simulink model "L4_sim1"  (R2024b)
settings: Solver=VariableStepAuto  StartTime=0.0  StopTime=100  RelTol=1e-3
values from neighbouring files (symbols this model uses):
  A_0 = eye(3)    [Task1.m]
  I = diag([Ix, Iy, Iz])    [Task1.m]    (also in Task3.m)
  orthonormalize = 0    [Task1.m]
  w_0 = [0.45, 0.52, 0.55]'    [Task1.m]    (also in Task3.m = [0.3, 0.15, 0.6]')
libraries: matrix_library x1
settings Model: Creator=alejandromunozvazquez  LastModifiedBy=alejandromunozvazquez

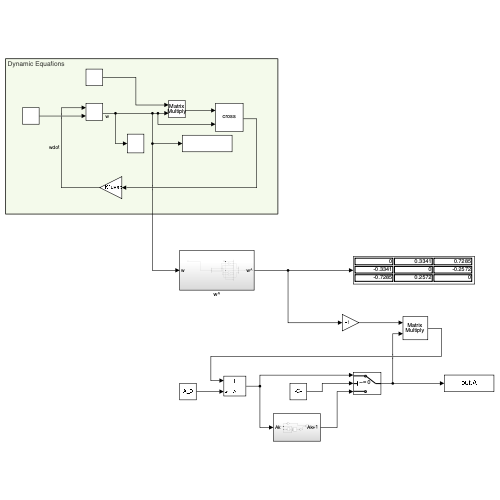
[thumbnail: Simulink's stored preview of the top-level diagram]
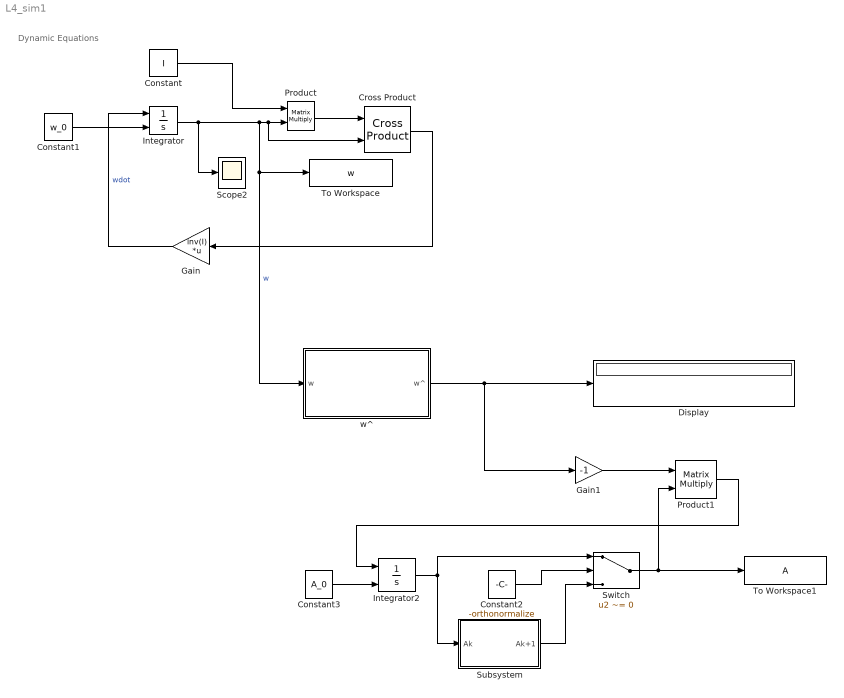
== system L4_sim1 ==
  note: Dynamic Equations
  Constant : Constant  Value=I
  Constant1 : Constant  Value=w_0
  Constant2 : Constant  Value=-orthonormalize
  Constant3 : Constant  Value=A_0
  Cross Product : matrix_library/Cross Product
  Display : Display
  Gain : Gain  Gain=inv(I)  Multiplication=Matrix(K*u) (u vector)
  Gain1 : Gain  Gain=-1
  Integrator : Integrator  InitialConditionSource=external
  Integrator2 : Integrator  InitialConditionSource=external
  Product : Product  Multiplication=Matrix(*)
  Product1 : Product  Multiplication=Matrix(*)
  Scope2 : Scope
  Subsystem : Subsystem
  Switch : Switch  Criteria=u2 ~= 0  SaturateOnIntegerOverflow=off  InputSameDT=off
  To Workspace : ToWorkspace  VariableName=w  SampleTime=-1
  To Workspace1 : ToWorkspace  VariableName=A  SampleTime=-1
  "w^ " : Subsystem
  wires:
  Gain/1 -> Integrator/1  "wdot"
  Integrator/1 -> Scope2/1, Product/2, Cross Product/2, "w^ "/1(w), To Workspace/1  "w"
  Constant/1 -> Product/1
  Product/1 -> Cross Product/1
  Cross Product/1 -> Gain/1
  Constant1/1 -> Integrator/2
  Product1/1 -> Integrator2/1
  Constant3/1 -> Integrator2/2
  Gain1/1 -> Product1/1
  Switch/1 -> Product1/2, To Workspace1/1
  "w^ "/1(w^) -> Gain1/1, Display/1
  Integrator2/1 -> Subsystem/1(Ak), Switch/1
  Subsystem/1(Ak+1) -> Switch/3
  Constant2/1 -> Switch/2

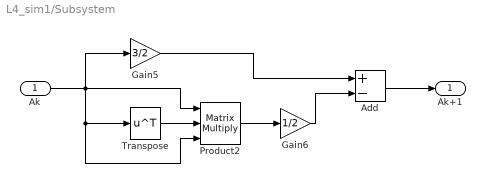
== system L4_sim1/Subsystem ==
  Ak : Inport
  Add : Sum  Inputs=+-
  Gain5 : Gain  Gain=3/2
  Gain6 : Gain  Gain=1/2
  Product2 : Product  Inputs=3  Multiplication=Matrix(*)
  Transpose : Math  Operator=transpose
  Ak+1 : Outport
  wires:
  Gain5/1 -> Add/1
  Add/1 -> Ak+1/1
  Product2/1 -> Gain6/1
  Gain6/1 -> Add/2
  Transpose/1 -> Product2/2
  Ak/1 -> Product2/3, Transpose/1, Gain5/1, Product2/1

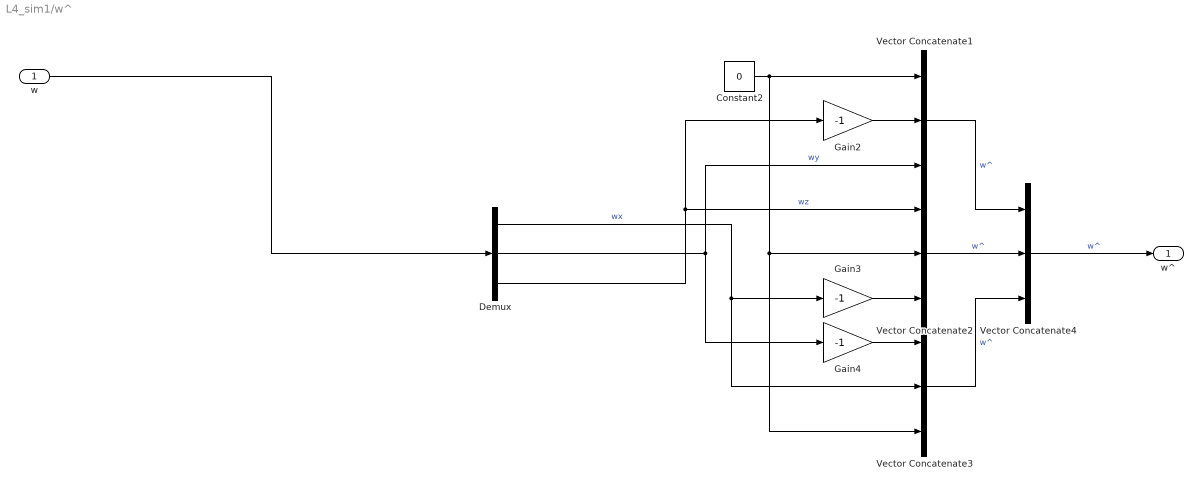
== system L4_sim1/w^  ==
  w : Inport
  Constant2 : Constant  Value=0
  Demux : Demux  Outputs=3
  Gain2 : Gain  Gain=-1
  Gain3 : Gain  Gain=-1
  Gain4 : Gain  Gain=-1
  Vector Concatenate1 : Concatenate  NumInputs=3  Mode=Multidimensional array
  Vector Concatenate2 : Concatenate  NumInputs=3  Mode=Multidimensional array
  Vector Concatenate3 : Concatenate  NumInputs=3  Mode=Multidimensional array
  Vector Concatenate4 : Concatenate  NumInputs=3  Mode=Multidimensional array  ConcatenateDimension=2
  w^ : Outport
  wires:
  w/1 -> Demux/1
  Vector Concatenate4/1 -> w^/1  "w^"
  Demux/2 -> Vector Concatenate1/3, Gain4/1  "wy"
  Vector Concatenate1/1 -> Vector Concatenate4/1  "w^"
  Demux/1 -> Vector Concatenate3/2, Gain3/1  "wx"
  Gain2/1 -> Vector Concatenate1/2
  Vector Concatenate3/1 -> Vector Concatenate4/3  "w^"
  Gain4/1 -> Vector Concatenate3/1
  Constant2/1 -> Vector Concatenate1/1, Vector Concatenate2/2, Vector Concatenate3/3
  Vector Concatenate2/1 -> Vector Concatenate4/2  "w^"
  Gain3/1 -> Vector Concatenate2/3
  Demux/3 -> Gain2/1, Vector Concatenate2/1  "wz"
